simulink model "patt"  (Simulink 6.4)
settings: Solver=FixedStepDiscrete  SolverMode=SingleTasking  StartTime=0.0  StopTime=20  RelTol=1e-3
InitFcn:
  | vipdh_pattern;
model workspace: external: M-Code (data not in the file)
values from neighbouring files (symbols this model uses):
  iut_dim = round([cat_info.Height cat_info.Width] * pyramiding_factor)    [vipdh_pattern.m]
  pyramiding_factor = 1/str2double(get_param(model_path,'pfactor'))    [vipdh_pattern.m]
  target_dim = size(target_img_pyramid)    [vipdh_pattern.m]
  target_dim_nopyramid = size(target_img)    [vipdh_pattern.m]
  target_fft = fftn(single(rot90(target_img_pyramid,2)),     [target_pad_rows target_pad_cols])    [vipdh_pattern.m]
  target_sq_sum = sqrt(sum(target_sq_sum(:)))    [vipdh_pattern.m]
undefined symbols (not defined in the file or in its folder): hot
libraries: vipsnks x2, viptextngfix x2, viptransforms x2, dspwin32 x1, vipmisc x1, vipstatistics x1, viputilities x1, dspmtrx3 x1, vipfilter x1, vipgeotforms x1, dspsnks4 x1
CloseFcn:
  | vipdh_pattern_clear;
settings Model: Creator=witek  LastModifiedBy=Administrator  ExtModeAutoUpdateStatusClock=off  ProdHWDeviceType=Specified
settings DataIOCC: LimitDataPoints=off  SaveOutput=off  SaveTime=off  SignalLoggingName=sigsOut
settings DebuggingCC: CheckExecutionContextPreStartOutputMsg=on  CheckExecutionContextRuntimeOutputMsg=on  SolverPrmCheckMsg=none  StrictBusMsg=None
settings HardwareCC: ProdHWDeviceType=Specified
settings ModelReferenceCC: UpdateModelReferenceTargets=IfOutOfDate

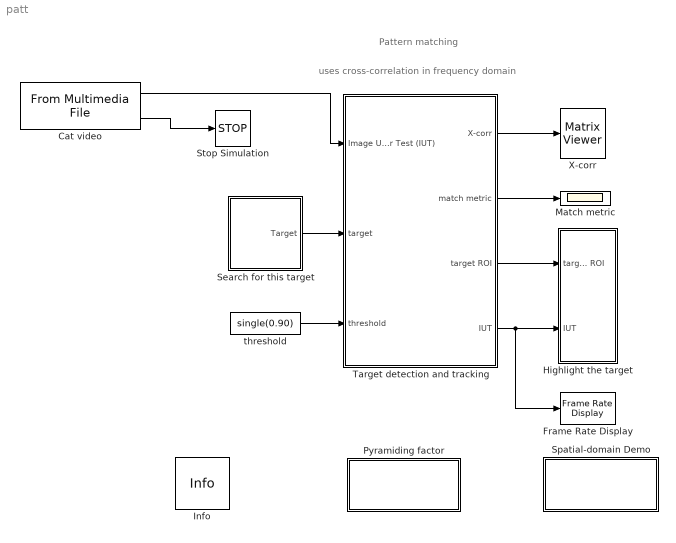
== system patt ==
  note: Pattern matching
  note: uses cross-correlation in frequency domain
  Cat video : dspwin32/From Multimedia File  DialogController=dspDDGCreate  DialogControllerArgs=DataTag0  inputFilename=C:\fypthings\things2.avi  loop=on  numPlays=inf  outputStreams=Video and audio  videoDataType=uint8  audioDataType=int16  inheritSampleTime=on  userDefinedSampleTime=1/30  noAudioOutput=off  isIntensityVideo=on  outputEOF=on
  Frame Rate Display : vipsnks/Frame Rate Display  DialogController=vipDDGCreate  DialogControllerArgs=DataTag1  UpdateRate=10
  Highlight the target : Subsystem
  Info : vipmisc/Info  SystemSampleTime=-1
  Match metric : Scope
      settings: TimeRange=10  YMin=0.75  YMax=1
  Pyramiding factor : Subsystem  mask(Pyramiding factor){pfactor=5}
      mask prompts: pfactor "Pyramiding factor"
      mask help:
      | The pyramiding factor is used to scale the input video so that the
      | cross-correlation is performed on a much smaller video frame thus
      | speeding up the pattern matching process.  The factor can be any
      | number from 1 to 5.  The accuracy of the match will degrade
      | proportionately to the size of the pyramiding factor.
      mask StyleString: popup(1|2|3|4|5)
      mask Display: disp('Set pyramiding\n factor')
  Search for this target : Subsystem
      mask Display: image(repmat(imread('things2_target.jpg'),[1,1,3]))
  Spatial-domain Demo : Subsystem
      settings: OpenFcn=patt_spat
      mask Type: Spatial-domain Demo
      mask Display: disp('Spatial-domain\nDemo')
  Stop Simulation : Stop
  Target detection and tracking : Subsystem
  X-corr : dspsnks4/Matrix Viewer  DialogController=dspdialog.MatrixViewer  DialogControllerArgs=DataTag9  ImageParams=on  CMapStr=hot(256)  AxisColorbar=on  AxisParams=on  AxisOrigin=Upper left corner  XLabel=X-axis  YLabel=Y-axis  ZLabel=Z-axis  FigPos=[578 341 369 234]  AxisZoom=off
      settings: YMin=0.7  YMax=1
  threshold : Constant  Value=single(0.90)  VectorParams1D=off  OutDataType=sfix(16)  ConRadixGroup=Use specified scaling  OutScaling=2^0  SampleTime=inf  FramePeriod=inf
  wires:
  Search for this target/1(Target) -> Target detection and tracking/2(target)
  Target detection and tracking/1(X-corr) -> X-corr/1
  Target detection and tracking/2(match metric) -> Match metric/1
  threshold/1 -> Target detection and tracking/3(threshold)
  Target detection and tracking/3(target ROI) -> Highlight the target/1(target ROI)
  Target detection and tracking/4(IUT) -> Highlight the target/2(IUT), Frame Rate Display/1
  Cat video/1 -> Target detection and tracking/1(Image Under Test (IUT))
  Cat video/2 -> Stop Simulation/1

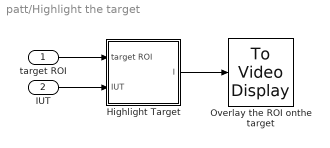
== system patt/Highlight the target ==
  target ROI : Inport
  IUT : Inport  Port=2
  Highlight Target : Subsystem
  Overlay the ROI onthe target : vipsnks/To Video Display  inputType=Intensity  OutputDevice=On-screen video monitor  fullScreen=off  videoWindowX=292  videoWindowY=157  saveWindowSize=off  videoWindowWidth=168  videoWindowHeight=147
  wires:
  Highlight Target/1(I) -> Overlay the ROI onthe target/1
  target ROI/1 -> Highlight Target/1(target ROI)
  IUT/1 -> Highlight Target/2(IUT)

== system patt/Pyramiding factor ==

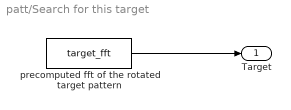
== system patt/Search for this target ==
  precomputed fft of the rotated target pattern : Constant  Value=target_fft  VectorParams1D=off  OutDataTypeMode=single  OutDataType=sfix(16)  ConRadixGroup=Use specified scaling  OutScaling=2^0  SampleTime=inf  FramePeriod=inf
  Target : Outport
  wires:
  precomputed fft of the rotated target pattern/1 -> Target/1

== system patt/Spatial-domain Demo ==

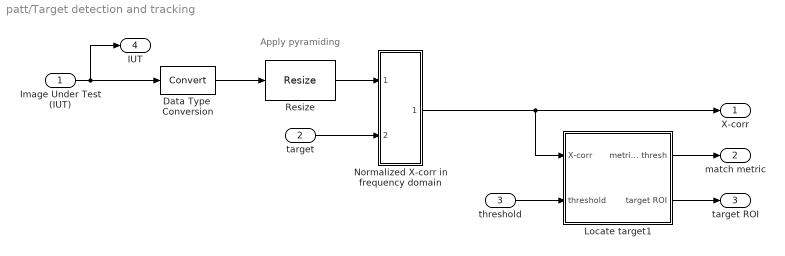
== system patt/Target detection and tracking ==
  note: Apply pyramiding
  Image Under Test (IUT) : Inport
  target : Inport  Port=2
  threshold : Inport  Port=3
  Data Type  Conversion : DataTypeConversion  OutDataTypeMode=single  SaturateOnIntegerOverflow=on  RndMeth=Zero
  Locate target1 : Subsystem
  Normalized X-corr in frequency domain : Subsystem
  Resize : vipgeotforms/Resize  DialogController=vipDDGCreate  DialogControllerArgs=DataTag8  specify=Output size as a percentage of input size  rfactor=pyramiding_factor*100  outCols=25  outRows=25  outRowsCols=[25 35]  interp_method=Bicubic  antialias=off  roundingMode=Floor  overflowMode=off
  X-corr : Outport
  match metric : Outport  Port=2
  target ROI : Outport  Port=3
  IUT : Outport  Port=4
  wires:
  target/1 -> Normalized X-corr in frequency domain/2(target)
  Image Under Test (IUT)/1 -> IUT/1, Data Type  Conversion/1
  Normalized X-corr in frequency domain/1(X-corr) -> X-corr/1, Locate target1/1(X-corr)
  Locate target1/2(target ROI) -> target ROI/1
  Locate target1/1(metric and thresh) -> match metric/1
  Data Type  Conversion/1 -> Resize/1
  threshold/1 -> Locate target1/2(threshold)
  Resize/1 -> Normalized X-corr in frequency domain/1(IUT)

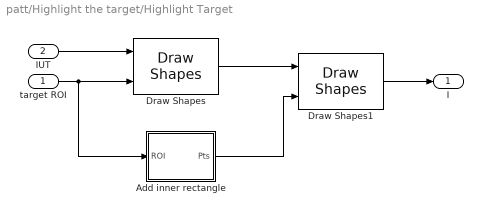
== system patt/Highlight the target/Highlight Target ==
  target ROI : Inport
  IUT : Inport  Port=2
  Add inner rectangle : Subsystem
  Draw Shapes : viptextngfix/Draw Shapes  DialogController=vipDDGCreate  DialogControllerArgs=DataTag2  inType=Intensity  shape=Rectangles  fill=off  display=Black  intensity=200  color=[200 255 100]  opacity=0.6  viewport=Entire image  antialiasing=off
  Draw Shapes1 : viptextngfix/Draw Shapes  DialogController=vipDDGCreate  DialogControllerArgs=DataTag3  inType=Intensity  shape=Rectangles  fill=off  display=White  intensity=200  color=[200 255 100]  opacity=0.6  viewport=Entire image  antialiasing=off
  I : Outport
  wires:
  IUT/1 -> Draw Shapes/1
  target ROI/1 -> Draw Shapes/2, Add inner rectangle/1(ROI)
  Add inner rectangle/1(Pts) -> Draw Shapes1/2
  Draw Shapes1/1 -> I/1
  Draw Shapes/1 -> Draw Shapes1/1

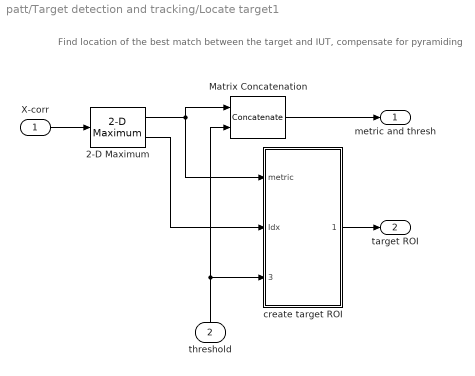
== system patt/Target detection and tracking/Locate target1 ==
  note: Find location of the best match
      | between the target and IUT,
      | compensate for pyramiding
  X-corr : Inport
  threshold : Inport  Orientation=up  Port=2
  2-D Maximum : vipstatistics/2-D Maximum  DialogController=dspDDGCreate  DialogControllerArgs=DataTag4  fcn=Value and Index  reset=None  roundingMode=Nearest  overflowMode=off
  Matrix Concatenation : Concatenate  Mode=Horizontal matrix concatenation
  create target ROI : Subsystem
  metric and thresh : Outport
  target ROI : Outport  Port=2
  wires:
  2-D Maximum/2 -> create target ROI/2(Idx)
  create target ROI/1(target ROI) -> target ROI/1
  X-corr/1 -> 2-D Maximum/1
  2-D Maximum/1 -> create target ROI/1(metric), Matrix Concatenation/1
  threshold/1 -> create target ROI/3(threshold), Matrix Concatenation/2
  Matrix Concatenation/1 -> metric and thresh/1

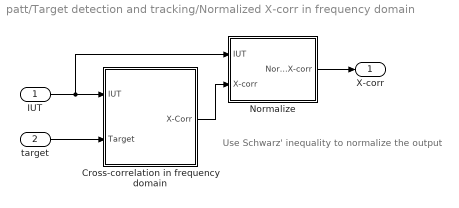
== system patt/Target detection and tracking/Normalized X-corr in frequency domain ==
  note: Use Schwarz' inequality
      | to normalize the output
  IUT : Inport
  target : Inport  Port=2
  Cross-correlation in frequency domain : Subsystem
  Normalize : Subsystem
  X-corr : Outport
  wires:
  Cross-correlation in frequency domain/1(X-Corr) -> Normalize/2(X-corr)
  IUT/1 -> Normalize/1(IUT), Cross-correlation in frequency domain/1(IUT)
  Normalize/1(Norm X-corr) -> X-corr/1
  target/1 -> Cross-correlation in frequency domain/2(Target)

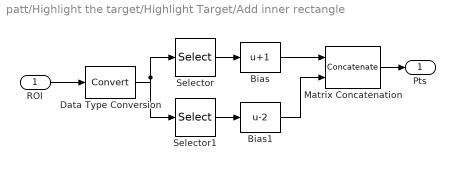
== system patt/Highlight the target/Highlight Target/Add inner rectangle ==
  ROI : Inport
  Bias : Bias  Bias=1
  Bias1 : Bias  Bias=-2
  Data Type Conversion : DataTypeConversion  OutDataTypeMode=int32
  Matrix Concatenation : Concatenate  Mode=Horizontal matrix concatenation
  Selector : Selector  IndexMode=Zero-based  Elements=[0 1]  InputPortWidth=4
  Selector1 : Selector  IndexMode=Zero-based  Elements=[2 3]  InputPortWidth=4
  Pts : Outport
  wires:
  Selector/1 -> Bias/1
  Selector1/1 -> Bias1/1
  Bias/1 -> Matrix Concatenation/1
  Bias1/1 -> Matrix Concatenation/2
  Data Type Conversion/1 -> Selector/1, Selector1/1
  ROI/1 -> Data Type Conversion/1
  Matrix Concatenation/1 -> Pts/1

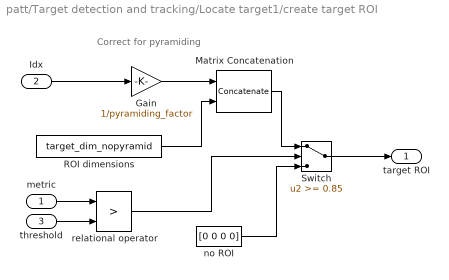
== system patt/Target detection and tracking/Locate target1/create target ROI ==
  note: Correct for
      |  pyramiding
  metric : Inport
  Idx : Inport  Port=2
  threshold : Inport  Port=3
  Gain : Gain  Gain=1/pyramiding_factor  ParameterDataTypeMode=Specify via dialog  ParameterDataType=float('single')  ParameterScalingMode=Best Precision: Element-wise  ParameterScaling=2^-16  RndMeth=Nearest  SaturateOnIntegerOverflow=on
  Matrix Concatenation : Concatenate  Mode=Horizontal matrix concatenation
  ROI dimensions : Constant  Value=target_dim_nopyramid  VectorParams1D=off  OutDataTypeMode=uint32  OutDataType=sfix(16)  ConRadixGroup=Use specified scaling  OutScaling=2^0  SampleTime=inf  FramePeriod=inf
  Switch : Switch  Threshold=0.85
  no ROI : Constant  Value=[0 0 0 0]  OutDataTypeMode=uint32  OutDataType=sfix(16)  ConRadixGroup=Use specified scaling  OutScaling=2^0  SampleTime=inf  FramePeriod=inf
  relational operator : RelationalOperator  Operator=>  LogicOutDataTypeMode=Boolean  ZeroCross=off
  target ROI : Outport
  wires:
  Idx/1 -> Gain/1
  Gain/1 -> Matrix Concatenation/1
  relational operator/1 -> Switch/2
  threshold/1 -> relational operator/2
  metric/1 -> relational operator/1
  no ROI/1 -> Switch/3
  Switch/1 -> target ROI/1
  ROI dimensions/1 -> Matrix Concatenation/2
  Matrix Concatenation/1 -> Switch/1

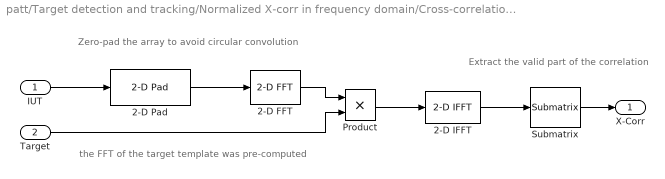
== system patt/Target detection and tracking/Normalized X-corr in frequency domain/Cross-correlation in frequency domain ==
  note: the FFT of the target template was pre-computed
  note: Zero-pad the array to avoid
      | circular convolution
  note: Extract the valid part
      | of the correlation
  IUT : Inport
  Target : Inport  Port=2
  2-D FFT : viptransforms/2-D FFT  DialogController=vipDDGCreate  DialogControllerArgs=DataTag5  TableOpt=Speed  BitRevOrder=off  SkipNorm=off  roundingMode=Floor  overflowMode=off
  2-D IFFT : viptransforms/2-D IFFT  DialogController=vipDDGCreate  DialogControllerArgs=DataTag6  SystemSampleTime=-1  TableOpt=Speed  BitRevOrder=off  cs_in=on  SkipNorm=off  roundingMode=Floor  overflowMode=off
  2-D Pad : viputilities/2-D Pad  method=Constant  valSrc=Specify via dialog  value=0  spec=Output size  rowDirection=Right  rowSize=2  outColSize=2^nextpow2(iut_dim(2)+target_dim(2)+1)  colDirection=Bottom  colSize=[2 3]  outRowSize=2^nextpow2(iut_dim(1)+target_dim(1)+1)
  Product : Product  RndMeth=Zero
  Submatrix : dspmtrx3/Submatrix  RowSpan=Range of rows  RowStartMode=Index  RowStartIndex=target_dim(1)  RowEndMode=Index  RowEndIndex=iut_dim(1)  ColSpan=Range of columns  ColStartMode=Index  ColStartIndex=target_dim(2)  ColEndMode=Index  ColEndIndex=iut_dim(2)
  X-Corr : Outport
  wires:
  Product/1 -> 2-D IFFT/1
  2-D FFT/1 -> Product/1
  2-D IFFT/1 -> Submatrix/1
  Submatrix/1 -> X-Corr/1
  IUT/1 -> 2-D Pad/1
  Target/1 -> Product/2
  2-D Pad/1 -> 2-D FFT/1

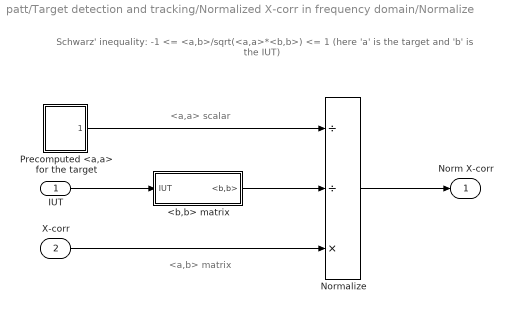
== system patt/Target detection and tracking/Normalized X-corr in frequency domain/Normalize ==
  note: Schwarz' inequality:
      | -1 <= <a,b>/sqrt(<a,a>*<b,b>) <= 1
      | (here 'a' is the target and 'b' is the IUT)
  note: <a,a> scalar
  note: <a,b> matrix
  IUT : Inport
  X-corr : Inport  Port=2
  <b,b> matrix : Subsystem
  Normalize : Product  Inputs=//*  SaturateOnIntegerOverflow=on  RndMeth=Zero
  Precomputed <a,a> for the target : Subsystem
      mask Display: image(repmat(imread('cat_target.png'),[1,1,3]))
  Norm X-corr : Outport
  wires:
  IUT/1 -> <b,b> matrix/1(IUT)
  Normalize/1 -> Norm X-corr/1
  <b,b> matrix/1(<b,b>) -> Normalize/2
  Precomputed <a,a> for the target/1(Target) -> Normalize/1
  X-corr/1 -> Normalize/3

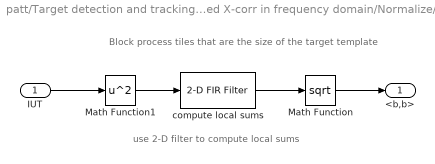
== system patt/Target detection and tracking/Normalized X-corr in frequency domain/Normalize/<b,b> matrix ==
  note: Block process tiles that are the size of the target template
  note: use 2-D filter to
      | compute local sums
  IUT : Inport
  Math Function : Math  Operator=sqrt  SaturateOnIntegerOverflow=on
  Math Function1 : Math  Operator=square  SaturateOnIntegerOverflow=on
  compute local sums : vipfilter/2-D FIR Filter  DialogController=vipDDGCreate  DialogControllerArgs=DataTag7  separable=off  filtSrc=Specify via dialog  filterMtrx=ones(target_dim)  verticalFilter=[4 0]  horizontalFilter=[4 0]  outSize=Valid  padType=Constant  padSrc=Specify via dialog  padVal=0  method=Convolution  roundingMode=Floor  overflowMode=off
  <b,b> : Outport
  wires:
  compute local sums/1 -> Math Function/1
  IUT/1 -> Math Function1/1
  Math Function1/1 -> compute local sums/1
  Math Function/1 -> <b,b>/1

== system patt/Target detection and tracking/Normalized X-corr in frequency domain/Normalize/Precomputed <a,a> for the target ==
  precomputed fft of the rotated target pattern : Constant  Value=target_sq_sum  VectorParams1D=off  OutDataTypeMode=single  OutDataType=sfix(16)  ConRadixGroup=Use specified scaling  OutScaling=2^0  SampleTime=inf  FramePeriod=inf
  Target : Outport
  wires:
  precomputed fft of the rotated target pattern/1 -> Target/1
